simulink model "RightTrajectoryAgent"  (Simulink 6.2)
settings: Solver=ode45  SolverMode=SingleTasking  StartTime=0.0  StopTime=10.0  RelTol=1e-3  AbsTol=1e-6
settings Model: Creator=The MathWorks Inc.  LastModifiedBy=suarezjl  ExtModeTrigMode=oneshot  ExtModeArmWhenConnect=off  ExtModeAutoUpdateStatusClock=off
settings DataIOCC: LimitDataPoints=off  SignalLoggingName=logsOut
settings OptimizationCC: BooleanDataType=off  InlineInvariantSignals=on
settings DebuggingCC: CheckExecutionContextPreStartOutputMsg=on  CheckExecutionContextRuntimeOutputMsg=on  IntegerOverflowMsg=none
settings HardwareCC: TargetUnknown=on
settings ModelReferenceCC: UpdateModelReferenceTargets=IfOutOfDate

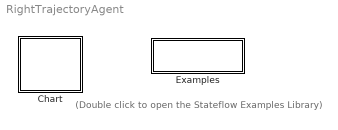
== system RightTrajectoryAgent ==
  note: (Double click to open the
      | Stateflow Examples Library)
  Chart : Stateflow chart
  Examples : Subsystem
      settings: OpenFcn=sf('Private','sf_examples')
      mask Display: disp('Examples')

== system RightTrajectoryAgent/Examples ==

== stateflow chart Chart ==
  state InitializeFunctions
    Popeye\RightTrajectoryAgent\LoadHomePosition.Initialize()
    Popeye\RightTrajectoryAgent\PlayCurrentTraj.Initialize()
    Popeye\RightTrajectoryAgent\LoadHomePosition.Write2VS()
  state CopyCurrentLocation
    Popeye\RightTrajectoryAgent\CopyGoalPosition.CopyRowVector()
    Popeye\RightTrajectoryAgent\CopyCurrentPosition.CopyCurrentVector()
  state GenerateCurrentTrajectory
    Popeye\RightTrajectoryAgent\GenerateCurrentTraj.GenerateTrajectory()
  state PlayCurrentTrajectory
    Popeye\RightTrajectoryAgent\PlayCurrentTraj.OutputTrajectory()
  state CopyHomeLocation
    Popeye\RightTrajectoryAgent\CopyHomePos.CopyRowVector()
    Popeye\RightTrajectoryAgent\CopyCurrentPosition.CopyCurrentVector()
  state PlayHomeTrajectory
    Popeye\RightTrajectoryAgent\PlayCurrentTraj.OutputTrajectory()
  state GenerateHomeTrajectory
    Popeye\RightTrajectoryAgent\GenerateCurrentTraj.GenerateTrajectory()
  (default) -> InitializeFunctions [order 1] : Start
  InitializeFunctions -> CopyCurrentLocation : Always
  CopyCurrentLocation -> GenerateCurrentTrajectory : Always
  (default) -> GenerateCurrentTrajectory [order 2] : Default
  GenerateCurrentTrajectory -> PlayCurrentTrajectory : Signal="Go to next state"
  PlayCurrentTrajectory -> PlayCurrentTrajectory [order 1] : Default
  PlayCurrentTrajectory -> CopyHomeLocation [order 2] : Always
  GenerateHomeTrajectory -> GenerateHomeTrajectory [order 1] : Default
  CopyHomeLocation -> GenerateHomeTrajectory : Always
  PlayHomeTrajectory -> PlayHomeTrajectory [order 1] : Default
  PlayHomeTrajectory -> CopyCurrentLocation [order 2] : Signal="Compute next trajectory"
  GenerateHomeTrajectory -> PlayHomeTrajectory [order 2] : Signal="Go to next state"
